simulink model "SegmentTransition"  (R2021b)
settings: Solver=VariableStepAuto  StartTime=0.0  StopTime=10.0  RelTol=1e-3
settings Model: DataDictionary=GuidanceDD.sldd  Creator=Paul  LastModifiedBy=Paul

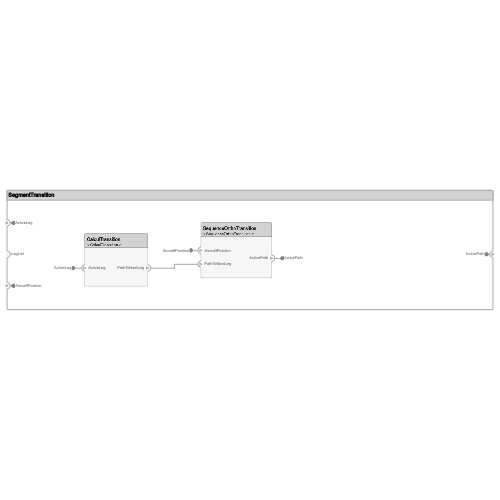
[thumbnail: Simulink's stored preview of the top-level diagram]
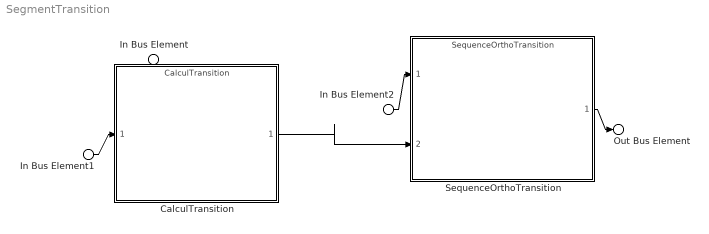
== system SegmentTransition ==
  In Bus Element1 : Inport  PortName=ActiveLeg
  In Bus Element : Inport  Port=2  PortName=LegList
  In Bus Element2 : Inport  Port=3  PortName=AircraftPosition
  CalculTransition : ModelReference  ModelNameDialog=CalculTransition  SimulationMode=Normal  ModelReferenceVersion=1.2
      settings: PortSchema="{\"entries\":[{\"content\":{\"headerSize\":38,\"margin\":15,\"minimumSpacing\":25,\"sides\":[{\"content\":{\"connectorIds\":[\"In1\"]},\"type\":\"ConnectorPlacement.EquallySpacedRectSide\",\"uuid\":\"eb69f848-a871-48e7-b646-0427db2d26df\"},{\"content\":{\"connectorIds\":[\"Out1\"],\"side\":\"RIGHT\"},\"type\":\"ConnectorPlacement.EquallySpacedRectSide\",\"uuid\":\"5e5c82fb-e123-44dd-bdc0-51d0c3877ae5\"},{\"content\":{\"connectorIds\":[],\"side\":\"TOP\"},\"type\":\"ConnectorPlacement.EquallySpacedRectSide\",\"uuid\":\"2dfda046-a579-4ba4-b882-f37fb2c038e7\"}]},\"type\":\"ConnectorPlacement.EquallySpacedConnector\",\"uuid\":\"2f3d76a7-403d-4fea-bddb-5280fa4ae833\"}],\"packageUris\":[\"http://schema.mathworks.com/mf0/Connector/R2020b\"],\"version\":\"1.0\"}"
  SequenceOrthoTransition : ModelReference  ModelNameDialog=SequenceOrthoTransition  SimulationMode=Normal  ModelReferenceVersion=1.2
      settings: PortSchema="{\"entries\":[{\"content\":{\"headerSize\":38,\"margin\":15,\"minimumSpacing\":25,\"sides\":[{\"content\":{\"connectorIds\":[\"In1\",\"In2\"]},\"type\":\"ConnectorPlacement.EquallySpacedRectSide\",\"uuid\":\"eb69f848-a871-48e7-b646-0427db2d26df\"},{\"content\":{\"connectorIds\":[\"Out1\"],\"side\":\"RIGHT\"},\"type\":\"ConnectorPlacement.EquallySpacedRectSide\",\"uuid\":\"5e5c82fb-e123-44dd-bdc0-51d0c3877ae5\"},{\"content\":{\"connectorIds\":[],\"side\":\"TOP\"},\"type\":\"ConnectorPlacement.EquallySpacedRectSide\",\"uuid\":\"2dfda046-a579-4ba4-b882-f37fb2c038e7\"}]},\"type\":\"ConnectorPlacement.EquallySpacedConnector\",\"uuid\":\"2f3d76a7-403d-4fea-bddb-5280fa4ae833\"}],\"packageUris\":[\"http://schema.mathworks.com/mf0/Connector/R2020b\"],\"version\":\"1.0\"}"
  Out Bus Element : Outport  PortName=ActivePath
  wires:
  In Bus Element1/1 -> CalculTransition/1
  In Bus Element2/1 -> SequenceOrthoTransition/1
  CalculTransition/1 -> SequenceOrthoTransition/2
  SequenceOrthoTransition/1 -> Out Bus Element/1
